simulink model "IEEE39_IBR_FrequencyControl_Primary_2020b"  (R2020b)
settings: Solver=VariableStepAuto  StartTime=0.0  StopTime=30  RelTol=1e-3
InitFcn:
  | IEEE39data_FrencyControl_primary;
undefined symbols (not defined in the file): Fref, IBR_data, line, Sbase, t_start_disturbance, Vbase
libraries: powerlib x203, powerlib_meascontrol x81, powerlib_extras x27, pid_lib x14
(part 2 of 5)

== system IEEE39_IBR_FrequencyControl_Primary_2020b/Subsystem ==
  Mux : Mux  Inputs=10
  Mux2 : Mux  Inputs=10
  Scope2 : Scope
  Scope3 : Scope
  wires:
  [f10] -> Mux/10
  [f1] -> Mux/1
  [f2] -> Mux/2
  [f3] -> Mux/3
  [f4] -> Mux/4
  [f5] -> Mux/5
  [f6] -> Mux/6
  [f7] -> Mux/7
  [f8] -> Mux/8
  [f9] -> Mux/9
  Mux/1 -> Scope2/1
  [P_GFL1] -> Mux2/1
  Mux2/1 -> Scope3/1
  [P_GFL2] -> Mux2/2
  [P_GFL3] -> Mux2/3
  [P_GFL4] -> Mux2/4
  [P_GFL5] -> Mux2/5
  [P_GFL6] -> Mux2/6
  [P_GFM7] -> Mux2/7
  [P_GFM8] -> Mux2/8
  [P_GFM9] -> Mux2/9
  [P_GFM10] -> Mux2/10

== system IEEE39_IBR_FrequencyControl_Primary_2020b/Bus voltages/V_F_measurements30 ==
  abc : Inport
  Display16 : Display
      settings: Format=bank
  PLL (3ph) : powerlib_meascontrol/PLL/PLL (3ph)  Fmin=59.5  Par_Init=[0, 60]  ParK=[180, 3200, 1]  TcD=1e-4  MaxRateChangeFreq=12  FilterCutOffFreq=25  Ts=1e-5  AGC=on
  tag scope: f1=global, f_B30=global
  wires:
  abc/1 -> PLL (3ph)/1
  PLL (3ph)/1 -> [f1], [f_B30], Display16/1

== system IEEE39_IBR_FrequencyControl_Primary_2020b/Bus voltages/V_F_measurements31 ==
  abc : Inport
  PLL (3ph) : powerlib_meascontrol/PLL/PLL (3ph)  Fmin=59.5  Par_Init=[0, 60]  ParK=[180, 3200, 1]  TcD=1e-4  MaxRateChangeFreq=12  FilterCutOffFreq=25  Ts=1e-5  AGC=on
  tag scope: f2=global, f_B31=global
  wires:
  abc/1 -> PLL (3ph)/1
  PLL (3ph)/1 -> [f2], [f_B31]

== system IEEE39_IBR_FrequencyControl_Primary_2020b/Bus voltages/V_F_measurements32 ==
  abc : Inport
  Display16 : Display
      settings: Format=bank
  PLL (3ph) : powerlib_meascontrol/PLL/PLL (3ph)  Fmin=59.5  Par_Init=[0, 60]  ParK=[180, 3200, 1]  TcD=1e-4  MaxRateChangeFreq=12  FilterCutOffFreq=25  Ts=1e-5  AGC=on
  tag scope: f3=global, f_B32=global
  wires:
  abc/1 -> PLL (3ph)/1
  PLL (3ph)/1 -> [f3], [f_B32], Display16/1

== system IEEE39_IBR_FrequencyControl_Primary_2020b/Bus voltages/V_F_measurements33 ==
  abc : Inport
  Display16 : Display
      settings: Format=bank
  PLL (3ph) : powerlib_meascontrol/PLL/PLL (3ph)  Fmin=59.5  Par_Init=[0, 60]  ParK=[180, 3200, 1]  TcD=1e-4  MaxRateChangeFreq=12  FilterCutOffFreq=25  Ts=1e-5  AGC=on
  tag scope: f4=global, f_B33=global
  wires:
  abc/1 -> PLL (3ph)/1
  PLL (3ph)/1 -> [f_B33], Display16/1, [f4]

== system IEEE39_IBR_FrequencyControl_Primary_2020b/Bus voltages/V_F_measurements34 ==
  abc : Inport
  Display16 : Display
      settings: Format=bank
  PLL (3ph) : powerlib_meascontrol/PLL/PLL (3ph)  Fmin=59.5  Par_Init=[0, 60]  ParK=[180, 3200, 1]  TcD=1e-4  MaxRateChangeFreq=12  FilterCutOffFreq=25  Ts=1e-5  AGC=on
  tag scope: f5=global, f_B34=global
  wires:
  abc/1 -> PLL (3ph)/1
  PLL (3ph)/1 -> [f_B34], Display16/1, [f5]

== system IEEE39_IBR_FrequencyControl_Primary_2020b/Bus voltages/V_F_measurements35 ==
  abc : Inport
  Display16 : Display
      settings: Format=bank
  PLL (3ph) : powerlib_meascontrol/PLL/PLL (3ph)  Fmin=59.5  Par_Init=[0, 60]  ParK=[180, 3200, 1]  TcD=1e-4  MaxRateChangeFreq=12  FilterCutOffFreq=25  Ts=1e-5  AGC=on
  tag scope: f6=global, f_B35=global
  wires:
  abc/1 -> PLL (3ph)/1
  PLL (3ph)/1 -> [f6], [f_B35], Display16/1

== system IEEE39_IBR_FrequencyControl_Primary_2020b/Bus voltages/V_F_measurements36 ==
  abc : Inport
  Display16 : Display
      settings: Format=bank
  PLL (3ph) : powerlib_meascontrol/PLL/PLL (3ph)  Fmin=59.5  Par_Init=[0, 60]  ParK=[180, 3200, 1]  TcD=1e-4  MaxRateChangeFreq=12  FilterCutOffFreq=25  Ts=1e-5  AGC=on
  tag scope: f7=global, f_B36=global
  wires:
  abc/1 -> PLL (3ph)/1
  PLL (3ph)/1 -> [f7], [f_B36], Display16/1

== system IEEE39_IBR_FrequencyControl_Primary_2020b/Bus voltages/V_F_measurements37 ==
  abc : Inport
  Display16 : Display
      settings: Format=bank
  PLL (3ph) : powerlib_meascontrol/PLL/PLL (3ph)  Fmin=59.5  Par_Init=[0, 60]  ParK=[180, 3200, 1]  TcD=1e-4  MaxRateChangeFreq=12  FilterCutOffFreq=25  Ts=1e-5  AGC=on
  tag scope: f8=global, f_B37=global
  wires:
  abc/1 -> PLL (3ph)/1
  PLL (3ph)/1 -> [f8], [f_B37], Display16/1

== system IEEE39_IBR_FrequencyControl_Primary_2020b/Bus voltages/V_F_measurements38 ==
  abc : Inport
  Display16 : Display
      settings: Format=bank
  PLL (3ph) : powerlib_meascontrol/PLL/PLL (3ph)  Fmin=59.5  Par_Init=[0, 60]  ParK=[180, 3200, 1]  TcD=1e-4  MaxRateChangeFreq=12  FilterCutOffFreq=25  Ts=1e-5  AGC=on
  tag scope: f9=global, f_B38=global
  wires:
  abc/1 -> PLL (3ph)/1
  PLL (3ph)/1 -> [f9], [f_B38], Display16/1

== system IEEE39_IBR_FrequencyControl_Primary_2020b/Bus voltages/V_F_measurements39 ==
  abc : Inport
  Display16 : Display
      settings: Format=bank
  PLL (3ph) : powerlib_meascontrol/PLL/PLL (3ph)  Fmin=59.5  Par_Init=[0, 60]  ParK=[180, 3200, 1]  TcD=1e-4  MaxRateChangeFreq=12  FilterCutOffFreq=25  Ts=1e-5  AGC=on
  tag scope: f10=global, f_B39=global
  wires:
  abc/1 -> PLL (3ph)/1
  PLL (3ph)/1 -> [f10], [f_B39], Display16/1

== system IEEE39_IBR_FrequencyControl_Primary_2020b/G1_GFL/PV_PQ3 ==
  Pref : Inport
  Qref : Inport  Port=2
  Fref : Inport  Port=3
  D : Inport  Port=4
  3-phase Instantaneous Active & Reactive Power4 : powerlib_extras/Measurements/3-phase  Instantaneous  Active & Reactive Power
  Controlled Voltage Source : powerlib/Electrical Sources/Controlled Voltage Source  Initialize=off  Source_Type=AC  Amplitude=0  Phase=0  Frequency=60  Measurements=None
  Controlled Voltage Source1 : powerlib/Electrical Sources/Controlled Voltage Source  Initialize=off  Source_Type=AC  Amplitude=0  Phase=-120  Frequency=60  Measurements=None
  Controlled Voltage Source3 : powerlib/Electrical Sources/Controlled Voltage Source  Initialize=off  Source_Type=DC  Amplitude=0  Phase=120  Frequency=60  Measurements=None
  Demux : Demux  Outputs=2
  Freq_Droop : Subsystem
  Ground : powerlib/Elements/Ground  LConnTagsString=a
  Ground1 : powerlib/Elements/Ground  LConnTagsString=a
  L : powerlib/Elements/Three-Phase Series RLC Branch  LConnTagsString=A|B|C  RConnTagsString=A|B|C  BranchType=RL  Resistance=0  Inductance=10e-3  Capacitance=1.0  Measurements=None
  L1 : Constant  Value=10e-3
  Mean : powerlib_meascontrol/Measurements/Mean  Freq=60  Vinit=0  Ts=5e-4
  PLL (3ph) : powerlib_meascontrol/PLL/PLL (3ph)  Fmin=59.5  Par_Init=[0, 60]  ParK=[180, 3200, 1]  TcD=1e-4  MaxRateChangeFreq=12  FilterCutOffFreq=25  Ts=1e-5  AGC=on
  Subsystem2 : Subsystem
  Terminator : Terminator
  Terminator1 : Terminator
  Three-Phase Series RLC Branch : powerlib/Elements/Three-Phase Series RLC Branch  LConnTagsString=A|B|C  RConnTagsString=A|B|C  BranchType=RC  Resistance=1000000  Inductance=1e-3  Capacitance=1000e-6  Measurements=None
  Three-Phase V-I Measurement : powerlib/Measurements/Three-Phase V-I Measurement  VoltageMeasurement=phase-to-ground  SetLabelV=off  LabelV=Vabc  Vpu=off  VpuLL=off  CurrentMeasurement=yes  SetLabelI=off  LabelI=Iabc  Ipu=off  Pbase=1e5  Vbase=380  OutputType=Complex  PhasorSimulation=off  PSBequivalent=0
  Three-Phase V-I Measurement4 : powerlib/Measurements/Three-Phase V-I Measurement  VoltageMeasurement=no  SetLabelV=off  LabelV=u  Vpu=off  VpuLL=off  CurrentMeasurement=yes  SetLabelI=off  LabelI=iFabcp3  Ipu=off  Pbase=100e6  Vbase=500e3  OutputType=Complex  PhasorSimulation=off  PSBequivalent=0
  Unit Delay : UnitDelay  SampleTime=-1  HasFrameUpgradeWarning=on
  Unit Delay1 : UnitDelay  SampleTime=-1  HasFrameUpgradeWarning=on
  Unit Delay2 : UnitDelay  SampleTime=-1  HasFrameUpgradeWarning=on
  PV_BatteryA : PMIOPort  Side=Right
  PV_BatteryB : PMIOPort  Port=2  Side=Right
  PV_BatteryC : PMIOPort  Port=3  Side=Right
  tag scope: P_GFL1=global
  wires:
  Three-Phase V-I Measurement/1 -> 3-phase Instantaneous Active & Reactive Power4/1, PLL (3ph)/1, Subsystem2/1(Vabcp)
  Three-Phase V-I Measurement/2 -> Subsystem2/2(Iabcp), 3-phase Instantaneous Active & Reactive Power4/2
  Mean/1 -> Demux/1
  L1/1 -> Subsystem2/6(L1)
  Three-Phase V-I Measurement4/1 -> Subsystem2/3(IFabcp)
  3-phase Instantaneous Active & Reactive Power4/1 -> Mean/1
  Qref/1 -> Subsystem2/5(Q_set)
  PLL (3ph)/2 -> Terminator/1
  PLL (3ph)/1 -> [Freq]
  Pref/1 -> Freq_Droop/1(Pref)
  Fref/1 -> Freq_Droop/2(Fref)
  [Freq] -> Freq_Droop/3(Freq)
  D/1 -> Freq_Droop/4(D)
  Freq_Droop/1(Pset) -> Subsystem2/4(P_set)
  Subsystem2/1(Va) -> Unit Delay/1
  Unit Delay/1 -> Controlled Voltage Source/1
  Subsystem2/2(Vb) -> Unit Delay1/1
  Unit Delay1/1 -> Controlled Voltage Source1/1
  Subsystem2/3(Vc) -> Unit Delay2/1
  Unit Delay2/1 -> Controlled Voltage Source3/1
  Demux/1 -> [P_GFL1]
  Demux/2 -> Terminator1/1
  connections:
  Three-Phase V-I Measurement/LConn1 -- Three-Phase Series RLC Branch/LConn1 -- L/RConn1
  Three-Phase V-I Measurement/RConn2 -- PV_BatteryB/RConn1
  Three-Phase V-I Measurement/LConn2 -- Three-Phase Series RLC Branch/LConn2 -- L/RConn2
  Three-Phase V-I Measurement4/LConn2 -- Controlled Voltage Source1/RConn1
  Controlled Voltage Source/RConn1 -- Three-Phase V-I Measurement4/LConn1
  Three-Phase V-I Measurement4/LConn3 -- Controlled Voltage Source3/RConn1
  Three-Phase V-I Measurement/LConn3 -- Three-Phase Series RLC Branch/LConn3 -- L/RConn3
  Three-Phase V-I Measurement/RConn3 -- PV_BatteryC/RConn1
  Three-Phase V-I Measurement/RConn1 -- PV_BatteryA/RConn1
  Three-Phase V-I Measurement4/RConn1 -- L/LConn1
  Three-Phase V-I Measurement4/RConn2 -- L/LConn2
  Three-Phase V-I Measurement4/RConn3 -- L/LConn3
  Three-Phase Series RLC Branch/RConn1 -- Ground1/LConn1 -- Three-Phase Series RLC Branch/RConn2 -- Three-Phase Series RLC Branch/RConn3
  Controlled Voltage Source/LConn1 -- Controlled Voltage Source3/LConn1 -- Controlled Voltage Source1/LConn1 -- Ground/LConn1

== system IEEE39_IBR_FrequencyControl_Primary_2020b/G2_GFL/PV_PQ3 ==
  Pref : Inport
  Qref : Inport  Port=2
  Fref : Inport  Port=3
  D : Inport  Port=4
  3-phase Instantaneous Active & Reactive Power4 : powerlib_extras/Measurements/3-phase  Instantaneous  Active & Reactive Power
  Controlled Voltage Source : powerlib/Electrical Sources/Controlled Voltage Source  Initialize=on  Source_Type=AC  Amplitude=391.87  Phase=0  Frequency=60  Measurements=None
  Controlled Voltage Source1 : powerlib/Electrical Sources/Controlled Voltage Source  Initialize=on  Source_Type=AC  Amplitude=391.87  Phase=-120  Frequency=60  Measurements=None
  Controlled Voltage Source3 : powerlib/Electrical Sources/Controlled Voltage Source  Initialize=on  Source_Type=AC  Amplitude=391.87  Phase=120  Frequency=60  Measurements=None
  Demux : Demux  Outputs=2
  Freq_Droop : Subsystem
  Ground : powerlib/Elements/Ground  LConnTagsString=a
  Ground1 : powerlib/Elements/Ground  LConnTagsString=a
  L : powerlib/Elements/Three-Phase Series RLC Branch  LConnTagsString=A|B|C  RConnTagsString=A|B|C  BranchType=RL  Resistance=0  Inductance=10e-3  Capacitance=1.0  Measurements=None
  L1 : Constant  Value=10e-3
  Mean : powerlib_meascontrol/Measurements/Mean  Freq=60  Vinit=0  Ts=5e-4
  PLL (3ph) : powerlib_meascontrol/PLL/PLL (3ph)  Fmin=59.5  Par_Init=[0, 60]  ParK=[180, 3200, 1]  TcD=1e-4  MaxRateChangeFreq=12  FilterCutOffFreq=25  Ts=1e-5  AGC=on
  Subsystem2 : Subsystem
  Terminator : Terminator
  Terminator1 : Terminator
  Three-Phase Series RLC Branch : powerlib/Elements/Three-Phase Series RLC Branch  LConnTagsString=A|B|C  RConnTagsString=A|B|C  BranchType=RC  Resistance=1000000  Inductance=1e-3  Capacitance=10000e-6  Measurements=None
  Three-Phase V-I Measurement : powerlib/Measurements/Three-Phase V-I Measurement  VoltageMeasurement=phase-to-ground  SetLabelV=off  LabelV=Vabc  Vpu=off  VpuLL=off  CurrentMeasurement=yes  SetLabelI=off  LabelI=Iabc  Ipu=off  Pbase=1e5  Vbase=380  OutputType=Complex  PhasorSimulation=off  PSBequivalent=0
  Three-Phase V-I Measurement4 : powerlib/Measurements/Three-Phase V-I Measurement  VoltageMeasurement=no  SetLabelV=off  LabelV=u  Vpu=off  VpuLL=off  CurrentMeasurement=yes  SetLabelI=off  LabelI=iFabcp3  Ipu=off  Pbase=100e6  Vbase=500e3  OutputType=Complex  PhasorSimulation=off  PSBequivalent=0
  Unit Delay : UnitDelay  SampleTime=-1  HasFrameUpgradeWarning=on
  Unit Delay1 : UnitDelay  SampleTime=-1  HasFrameUpgradeWarning=on
  Unit Delay2 : UnitDelay  SampleTime=-1  HasFrameUpgradeWarning=on
  PV_BatteryA : PMIOPort  Side=Right
  PV_BatteryB : PMIOPort  Port=2  Side=Right
  PV_BatteryC : PMIOPort  Port=3  Side=Right
  tag scope: P_GFL2=global
  wires:
  Three-Phase V-I Measurement/1 -> 3-phase Instantaneous Active & Reactive Power4/1, PLL (3ph)/1, Subsystem2/1(Vabcp)
  Three-Phase V-I Measurement/2 -> Subsystem2/2(Iabcp), 3-phase Instantaneous Active & Reactive Power4/2
  L1/1 -> Subsystem2/6(L1)
  Three-Phase V-I Measurement4/1 -> Subsystem2/3(IFabcp)
  3-phase Instantaneous Active & Reactive Power4/1 -> Mean/1
  Qref/1 -> Subsystem2/5(Q_set)
  PLL (3ph)/2 -> Terminator/1
  PLL (3ph)/1 -> [Freq]
  Pref/1 -> Freq_Droop/1(Pref)
  Fref/1 -> Freq_Droop/2(Fref)
  [Freq] -> Freq_Droop/3(Freq)
  D/1 -> Freq_Droop/4(D)
  Freq_Droop/1(Pset) -> Subsystem2/4(P_set)
  Subsystem2/1(Va) -> Unit Delay/1
  Unit Delay/1 -> Controlled Voltage Source/1
  Subsystem2/2(Vb) -> Unit Delay1/1
  Unit Delay1/1 -> Controlled Voltage Source1/1
  Subsystem2/3(Vc) -> Unit Delay2/1
  Unit Delay2/1 -> Controlled Voltage Source3/1
  Demux/2 -> Terminator1/1
  Demux/1 -> [P_GFL2]
  Mean/1 -> Demux/1
  connections:
  Three-Phase V-I Measurement/LConn1 -- Three-Phase Series RLC Branch/LConn1 -- L/RConn1
  Three-Phase V-I Measurement/RConn2 -- PV_BatteryB/RConn1
  Three-Phase V-I Measurement/LConn2 -- Three-Phase Series RLC Branch/LConn2 -- L/RConn2
  Three-Phase V-I Measurement4/LConn2 -- Controlled Voltage Source1/RConn1
  Controlled Voltage Source/RConn1 -- Three-Phase V-I Measurement4/LConn1
  Three-Phase V-I Measurement4/LConn3 -- Controlled Voltage Source3/RConn1
  Three-Phase V-I Measurement/LConn3 -- Three-Phase Series RLC Branch/LConn3 -- L/RConn3
  Three-Phase V-I Measurement/RConn3 -- PV_BatteryC/RConn1
  Three-Phase V-I Measurement/RConn1 -- PV_BatteryA/RConn1
  Three-Phase V-I Measurement4/RConn1 -- L/LConn1
  Three-Phase V-I Measurement4/RConn2 -- L/LConn2
  Three-Phase V-I Measurement4/RConn3 -- L/LConn3
  Three-Phase Series RLC Branch/RConn1 -- Ground1/LConn1 -- Three-Phase Series RLC Branch/RConn2 -- Three-Phase Series RLC Branch/RConn3
  Controlled Voltage Source/LConn1 -- Controlled Voltage Source3/LConn1 -- Controlled Voltage Source1/LConn1 -- Ground/LConn1

== system IEEE39_IBR_FrequencyControl_Primary_2020b/G3_GFL/PV_PQ3 ==
  Pref : Inport
  Qref : Inport  Port=2
  Fref : Inport  Port=3
  D : Inport  Port=4
  3-phase Instantaneous Active & Reactive Power4 : powerlib_extras/Measurements/3-phase  Instantaneous  Active & Reactive Power
  Controlled Voltage Source : powerlib/Electrical Sources/Controlled Voltage Source  Initialize=on  Source_Type=AC  Amplitude=391.87  Phase=0  Frequency=60  Measurements=None
  Controlled Voltage Source1 : powerlib/Electrical Sources/Controlled Voltage Source  Initialize=on  Source_Type=AC  Amplitude=391.87  Phase=-120  Frequency=60  Measurements=None
  Controlled Voltage Source3 : powerlib/Electrical Sources/Controlled Voltage Source  Initialize=on  Source_Type=AC  Amplitude=391.87  Phase=120  Frequency=60  Measurements=None
  Demux : Demux  Outputs=2
  Freq_Droop : Subsystem
  Ground : powerlib/Elements/Ground  LConnTagsString=a
  Ground1 : powerlib/Elements/Ground  LConnTagsString=a
  L : powerlib/Elements/Three-Phase Series RLC Branch  LConnTagsString=A|B|C  RConnTagsString=A|B|C  BranchType=RL  Resistance=0  Inductance=100e-3  Capacitance=1.0  Measurements=None
  L1 : Constant  Value=100e-3
  Mean : powerlib_meascontrol/Measurements/Mean  Freq=60  Vinit=0  Ts=5e-4
  PLL (3ph) : powerlib_meascontrol/PLL/PLL (3ph)  Fmin=59.5  Par_Init=[0, 60]  ParK=[180, 3200, 1]  TcD=1e-4  MaxRateChangeFreq=12  FilterCutOffFreq=25  Ts=1e-5  AGC=on
  Subsystem2 : Subsystem
  Terminator : Terminator
  Terminator1 : Terminator
  Three-Phase Series RLC Branch : powerlib/Elements/Three-Phase Series RLC Branch  LConnTagsString=A|B|C  RConnTagsString=A|B|C  BranchType=RC  Resistance=1000000  Inductance=1e-3  Capacitance=10000e-6  Measurements=None
  Three-Phase V-I Measurement : powerlib/Measurements/Three-Phase V-I Measurement  VoltageMeasurement=phase-to-ground  SetLabelV=off  LabelV=Vabc  Vpu=off  VpuLL=off  CurrentMeasurement=yes  SetLabelI=off  LabelI=Iabc  Ipu=off  Pbase=1e5  Vbase=380  OutputType=Complex  PhasorSimulation=off  PSBequivalent=0
  Three-Phase V-I Measurement4 : powerlib/Measurements/Three-Phase V-I Measurement  VoltageMeasurement=no  SetLabelV=off  LabelV=u  Vpu=off  VpuLL=off  CurrentMeasurement=yes  SetLabelI=off  LabelI=iFabcp3  Ipu=off  Pbase=100e6  Vbase=500e3  OutputType=Complex  PhasorSimulation=off  PSBequivalent=0
  Unit Delay : UnitDelay  SampleTime=-1  HasFrameUpgradeWarning=on
  Unit Delay1 : UnitDelay  SampleTime=-1  HasFrameUpgradeWarning=on
  Unit Delay2 : UnitDelay  SampleTime=-1  HasFrameUpgradeWarning=on
  PV_BatteryA : PMIOPort  Side=Right
  PV_BatteryB : PMIOPort  Port=2  Side=Right
  PV_BatteryC : PMIOPort  Port=3  Side=Right
  tag scope: P_GFL3=global
  wires:
  Three-Phase V-I Measurement/2 -> Subsystem2/2(Iabcp), 3-phase Instantaneous Active & Reactive Power4/2
  L1/1 -> Subsystem2/6(L1)
  Three-Phase V-I Measurement4/1 -> Subsystem2/3(IFabcp)
  3-phase Instantaneous Active & Reactive Power4/1 -> Mean/1
  Qref/1 -> Subsystem2/5(Q_set)
  Pref/1 -> Freq_Droop/1(Pref)
  Fref/1 -> Freq_Droop/2(Fref)
  [Freq] -> Freq_Droop/3(Freq)
  D/1 -> Freq_Droop/4(D)
  Freq_Droop/1(Pset) -> Subsystem2/4(P_set)
  Subsystem2/1(Va) -> Unit Delay/1
  Unit Delay/1 -> Controlled Voltage Source/1
  Subsystem2/2(Vb) -> Unit Delay1/1
  Unit Delay1/1 -> Controlled Voltage Source1/1
  Subsystem2/3(Vc) -> Unit Delay2/1
  Unit Delay2/1 -> Controlled Voltage Source3/1
  Demux/2 -> Terminator1/1
  Demux/1 -> [P_GFL3]
  Mean/1 -> Demux/1
  PLL (3ph)/2 -> Terminator/1
  PLL (3ph)/1 -> [Freq]
  Three-Phase V-I Measurement/1 -> PLL (3ph)/1, 3-phase Instantaneous Active & Reactive Power4/1, Subsystem2/1(Vabcp)
  connections:
  Three-Phase V-I Measurement/LConn1 -- Three-Phase Series RLC Branch/LConn1 -- L/RConn1
  Three-Phase V-I Measurement/RConn2 -- PV_BatteryB/RConn1
  Three-Phase V-I Measurement/LConn2 -- Three-Phase Series RLC Branch/LConn2 -- L/RConn2
  Three-Phase V-I Measurement4/LConn2 -- Controlled Voltage Source1/RConn1
  Controlled Voltage Source/RConn1 -- Three-Phase V-I Measurement4/LConn1
  Three-Phase V-I Measurement4/LConn3 -- Controlled Voltage Source3/RConn1
  Three-Phase V-I Measurement/LConn3 -- Three-Phase Series RLC Branch/LConn3 -- L/RConn3
  Three-Phase V-I Measurement/RConn3 -- PV_BatteryC/RConn1
  Three-Phase V-I Measurement/RConn1 -- PV_BatteryA/RConn1
  Three-Phase V-I Measurement4/RConn1 -- L/LConn1
  Three-Phase V-I Measurement4/RConn2 -- L/LConn2
  Three-Phase V-I Measurement4/RConn3 -- L/LConn3
  Three-Phase Series RLC Branch/RConn1 -- Ground1/LConn1 -- Three-Phase Series RLC Branch/RConn2 -- Three-Phase Series RLC Branch/RConn3
  Controlled Voltage Source/LConn1 -- Controlled Voltage Source3/LConn1 -- Controlled Voltage Source1/LConn1 -- Ground/LConn1

== system IEEE39_IBR_FrequencyControl_Primary_2020b/G4_GFL1/PV_PQ3 ==
  Pref : Inport
  Qref : Inport  Port=2
  Fref : Inport  Port=3
  D : Inport  Port=4
  3-phase Instantaneous Active & Reactive Power4 : powerlib_extras/Measurements/3-phase  Instantaneous  Active & Reactive Power
  Controlled Voltage Source : powerlib/Electrical Sources/Controlled Voltage Source  Initialize=on  Source_Type=AC  Amplitude=391.87  Phase=0  Frequency=60  Measurements=None
  Controlled Voltage Source1 : powerlib/Electrical Sources/Controlled Voltage Source  Initialize=on  Source_Type=AC  Amplitude=391.87  Phase=-120  Frequency=60  Measurements=None
  Controlled Voltage Source3 : powerlib/Electrical Sources/Controlled Voltage Source  Initialize=on  Source_Type=AC  Amplitude=391.87  Phase=120  Frequency=60  Measurements=None
  Demux : Demux  Outputs=2
  Freq_Droop : Subsystem
  Ground : powerlib/Elements/Ground  LConnTagsString=a
  Ground1 : powerlib/Elements/Ground  LConnTagsString=a
  L : powerlib/Elements/Three-Phase Series RLC Branch  LConnTagsString=A|B|C  RConnTagsString=A|B|C  BranchType=RL  Resistance=0  Inductance=10e-3  Capacitance=1.0  Measurements=None
  L1 : Constant  Value=10e-3
  Mean : powerlib_meascontrol/Measurements/Mean  Freq=60  Vinit=0  Ts=5e-4
  PLL (3ph) : powerlib_meascontrol/PLL/PLL (3ph)  Fmin=59.5  Par_Init=[0, 60]  ParK=[180, 3200, 1]  TcD=1e-4  MaxRateChangeFreq=12  FilterCutOffFreq=25  Ts=1e-5  AGC=on
  Subsystem2 : Subsystem
  Terminator : Terminator
  Terminator1 : Terminator
  Three-Phase Series RLC Branch : powerlib/Elements/Three-Phase Series RLC Branch  LConnTagsString=A|B|C  RConnTagsString=A|B|C  BranchType=RC  Resistance=1000000  Inductance=1e-3  Capacitance=100e-6  Measurements=None
  Three-Phase V-I Measurement : powerlib/Measurements/Three-Phase V-I Measurement  VoltageMeasurement=phase-to-ground  SetLabelV=off  LabelV=Vabc  Vpu=off  VpuLL=off  CurrentMeasurement=yes  SetLabelI=off  LabelI=Iabc  Ipu=off  Pbase=1e5  Vbase=380  OutputType=Complex  PhasorSimulation=off  PSBequivalent=0
  Three-Phase V-I Measurement4 : powerlib/Measurements/Three-Phase V-I Measurement  VoltageMeasurement=no  SetLabelV=off  LabelV=u  Vpu=off  VpuLL=off  CurrentMeasurement=yes  SetLabelI=off  LabelI=iFabcp3  Ipu=off  Pbase=100e6  Vbase=500e3  OutputType=Complex  PhasorSimulation=off  PSBequivalent=0
  Unit Delay : UnitDelay  SampleTime=-1  HasFrameUpgradeWarning=on
  Unit Delay1 : UnitDelay  SampleTime=-1  HasFrameUpgradeWarning=on
  Unit Delay2 : UnitDelay  SampleTime=-1  HasFrameUpgradeWarning=on
  PV_BatteryA : PMIOPort  Side=Right
  PV_BatteryB : PMIOPort  Port=2  Side=Right
  PV_BatteryC : PMIOPort  Port=3  Side=Right
  tag scope: P_GFL4=global
  wires:
  Three-Phase V-I Measurement/1 -> 3-phase Instantaneous Active & Reactive Power4/1, PLL (3ph)/1, Subsystem2/1(Vabcp)
  Three-Phase V-I Measurement/2 -> Subsystem2/2(Iabcp), 3-phase Instantaneous Active & Reactive Power4/2
  L1/1 -> Subsystem2/6(L1)
  Three-Phase V-I Measurement4/1 -> Subsystem2/3(IFabcp)
  3-phase Instantaneous Active & Reactive Power4/1 -> Mean/1
  Qref/1 -> Subsystem2/5(Q_set)
  PLL (3ph)/2 -> Terminator/1
  PLL (3ph)/1 -> [Freq]
  Pref/1 -> Freq_Droop/1(Pref)
  Fref/1 -> Freq_Droop/2(Fref)
  [Freq] -> Freq_Droop/3(Freq)
  D/1 -> Freq_Droop/4(D)
  Freq_Droop/1(Pset) -> Subsystem2/4(P_set)
  Subsystem2/1(Va) -> Unit Delay/1
  Unit Delay/1 -> Controlled Voltage Source/1
  Subsystem2/2(Vb) -> Unit Delay1/1
  Unit Delay1/1 -> Controlled Voltage Source1/1
  Subsystem2/3(Vc) -> Unit Delay2/1
  Unit Delay2/1 -> Controlled Voltage Source3/1
  Demux/2 -> Terminator1/1
  Demux/1 -> [P_GFL4]
  Mean/1 -> Demux/1
  connections:
  Three-Phase V-I Measurement/LConn1 -- Three-Phase Series RLC Branch/LConn1 -- L/RConn1
  Three-Phase V-I Measurement/RConn2 -- PV_BatteryB/RConn1
  Three-Phase V-I Measurement/LConn2 -- Three-Phase Series RLC Branch/LConn2 -- L/RConn2
  Three-Phase V-I Measurement4/LConn2 -- Controlled Voltage Source1/RConn1
  Controlled Voltage Source/RConn1 -- Three-Phase V-I Measurement4/LConn1
  Three-Phase V-I Measurement4/LConn3 -- Controlled Voltage Source3/RConn1
  Three-Phase V-I Measurement/LConn3 -- Three-Phase Series RLC Branch/LConn3 -- L/RConn3
  Three-Phase V-I Measurement/RConn3 -- PV_BatteryC/RConn1
  Three-Phase V-I Measurement/RConn1 -- PV_BatteryA/RConn1
  Three-Phase V-I Measurement4/RConn1 -- L/LConn1
  Three-Phase V-I Measurement4/RConn2 -- L/LConn2
  Three-Phase V-I Measurement4/RConn3 -- L/LConn3
  Three-Phase Series RLC Branch/RConn1 -- Ground1/LConn1 -- Three-Phase Series RLC Branch/RConn2 -- Three-Phase Series RLC Branch/RConn3
  Controlled Voltage Source/LConn1 -- Controlled Voltage Source3/LConn1 -- Controlled Voltage Source1/LConn1 -- Ground/LConn1

== system IEEE39_IBR_FrequencyControl_Primary_2020b/G5_GFL/PV_PQ3 ==
  Pref : Inport
  Qref : Inport  Port=2
  Fref : Inport  Port=3
  D : Inport  Port=4
  3-phase Instantaneous Active & Reactive Power4 : powerlib_extras/Measurements/3-phase  Instantaneous  Active & Reactive Power
  Controlled Voltage Source : powerlib/Electrical Sources/Controlled Voltage Source  Initialize=on  Source_Type=AC  Amplitude=391.87  Phase=0  Frequency=60  Measurements=None
  Controlled Voltage Source1 : powerlib/Electrical Sources/Controlled Voltage Source  Initialize=on  Source_Type=AC  Amplitude=391.87  Phase=-120  Frequency=60  Measurements=None
  Controlled Voltage Source3 : powerlib/Electrical Sources/Controlled Voltage Source  Initialize=on  Source_Type=AC  Amplitude=391.87  Phase=120  Frequency=60  Measurements=None
  Demux : Demux  Outputs=2
  Freq_Droop : Subsystem
  Ground : powerlib/Elements/Ground  LConnTagsString=a
  Ground1 : powerlib/Elements/Ground  LConnTagsString=a
  L : powerlib/Elements/Three-Phase Series RLC Branch  LConnTagsString=A|B|C  RConnTagsString=A|B|C  BranchType=RL  Resistance=0  Inductance=100e-3  Capacitance=1.0  Measurements=None
  L1 : Constant  Value=100e-3
  Mean : powerlib_meascontrol/Measurements/Mean  Freq=60  Vinit=0  Ts=5e-4
  PLL (3ph) : powerlib_meascontrol/PLL/PLL (3ph)  Fmin=59.5  Par_Init=[0, 60]  ParK=[180, 3200, 1]  TcD=1e-4  MaxRateChangeFreq=12  FilterCutOffFreq=25  Ts=1e-5  AGC=on
  Subsystem2 : Subsystem
  Terminator : Terminator
  Terminator1 : Terminator
  Three-Phase Series RLC Branch : powerlib/Elements/Three-Phase Series RLC Branch  LConnTagsString=A|B|C  RConnTagsString=A|B|C  BranchType=RC  Resistance=1000000  Inductance=1e-3  Capacitance=100e-6  Measurements=None
  Three-Phase V-I Measurement : powerlib/Measurements/Three-Phase V-I Measurement  VoltageMeasurement=phase-to-ground  SetLabelV=off  LabelV=Vabc  Vpu=off  VpuLL=off  CurrentMeasurement=yes  SetLabelI=off  LabelI=Iabc  Ipu=off  Pbase=1e5  Vbase=380  OutputType=Complex  PhasorSimulation=off  PSBequivalent=0
  Three-Phase V-I Measurement4 : powerlib/Measurements/Three-Phase V-I Measurement  VoltageMeasurement=no  SetLabelV=off  LabelV=u  Vpu=off  VpuLL=off  CurrentMeasurement=yes  SetLabelI=off  LabelI=iFabcp3  Ipu=off  Pbase=100e6  Vbase=500e3  OutputType=Complex  PhasorSimulation=off  PSBequivalent=0
  Unit Delay : UnitDelay  SampleTime=-1  HasFrameUpgradeWarning=on
  Unit Delay1 : UnitDelay  SampleTime=-1  HasFrameUpgradeWarning=on
  Unit Delay2 : UnitDelay  SampleTime=-1  HasFrameUpgradeWarning=on
  PV_BatteryA : PMIOPort  Side=Right
  PV_BatteryB : PMIOPort  Port=2  Side=Right
  PV_BatteryC : PMIOPort  Port=3  Side=Right
  tag scope: P_GFL5=global
  wires:
  Three-Phase V-I Measurement/1 -> 3-phase Instantaneous Active & Reactive Power4/1, PLL (3ph)/1, Subsystem2/1(Vabcp)
  Three-Phase V-I Measurement/2 -> Subsystem2/2(Iabcp), 3-phase Instantaneous Active & Reactive Power4/2
  L1/1 -> Subsystem2/6(L1)
  Three-Phase V-I Measurement4/1 -> Subsystem2/3(IFabcp)
  3-phase Instantaneous Active & Reactive Power4/1 -> Mean/1
  Qref/1 -> Subsystem2/5(Q_set)
  PLL (3ph)/2 -> Terminator/1
  PLL (3ph)/1 -> [Freq]
  Pref/1 -> Freq_Droop/1(Pref)
  Fref/1 -> Freq_Droop/2(Fref)
  [Freq] -> Freq_Droop/3(Freq)
  D/1 -> Freq_Droop/4(D)
  Freq_Droop/1(Pset) -> Subsystem2/4(P_set)
  Subsystem2/1(Va) -> Unit Delay/1
  Unit Delay/1 -> Controlled Voltage Source/1
  Subsystem2/2(Vb) -> Unit Delay1/1
  Unit Delay1/1 -> Controlled Voltage Source1/1
  Subsystem2/3(Vc) -> Unit Delay2/1
  Unit Delay2/1 -> Controlled Voltage Source3/1
  Demux/2 -> Terminator1/1
  Demux/1 -> [P_GFL5]
  Mean/1 -> Demux/1
  connections:
  Three-Phase V-I Measurement/LConn1 -- Three-Phase Series RLC Branch/LConn1 -- L/RConn1
  Three-Phase V-I Measurement/RConn2 -- PV_BatteryB/RConn1
  Three-Phase V-I Measurement/LConn2 -- Three-Phase Series RLC Branch/LConn2 -- L/RConn2
  Three-Phase V-I Measurement4/LConn2 -- Controlled Voltage Source1/RConn1
  Controlled Voltage Source/RConn1 -- Three-Phase V-I Measurement4/LConn1
  Three-Phase V-I Measurement4/LConn3 -- Controlled Voltage Source3/RConn1
  Three-Phase V-I Measurement/LConn3 -- Three-Phase Series RLC Branch/LConn3 -- L/RConn3
  Three-Phase V-I Measurement/RConn3 -- PV_BatteryC/RConn1
  Three-Phase V-I Measurement/RConn1 -- PV_BatteryA/RConn1
  Three-Phase V-I Measurement4/RConn1 -- L/LConn1
  Three-Phase V-I Measurement4/RConn2 -- L/LConn2
  Three-Phase V-I Measurement4/RConn3 -- L/LConn3
  Three-Phase Series RLC Branch/RConn1 -- Ground1/LConn1 -- Three-Phase Series RLC Branch/RConn2 -- Three-Phase Series RLC Branch/RConn3
  Controlled Voltage Source/LConn1 -- Controlled Voltage Source3/LConn1 -- Controlled Voltage Source1/LConn1 -- Ground/LConn1

== system IEEE39_IBR_FrequencyControl_Primary_2020b/G6_GFL/PV_PQ3 ==
  Pref : Inport
  Qref : Inport  Port=2
  Fref : Inport  Port=3
  D : Inport  Port=4
  3-phase Instantaneous Active & Reactive Power4 : powerlib_extras/Measurements/3-phase  Instantaneous  Active & Reactive Power
  Controlled Voltage Source : powerlib/Electrical Sources/Controlled Voltage Source  Initialize=on  Source_Type=AC  Amplitude=391.87  Phase=0  Frequency=60  Measurements=None
  Controlled Voltage Source1 : powerlib/Electrical Sources/Controlled Voltage Source  Initialize=on  Source_Type=AC  Amplitude=391.87  Phase=-120  Frequency=60  Measurements=None
  Controlled Voltage Source3 : powerlib/Electrical Sources/Controlled Voltage Source  Initialize=on  Source_Type=AC  Amplitude=391.87  Phase=120  Frequency=60  Measurements=None
  Demux : Demux  Outputs=2
  Freq_Droop : Subsystem
  Ground : powerlib/Elements/Ground  LConnTagsString=a
  Ground1 : powerlib/Elements/Ground  LConnTagsString=a
  L : powerlib/Elements/Three-Phase Series RLC Branch  LConnTagsString=A|B|C  RConnTagsString=A|B|C  BranchType=RL  Resistance=0  Inductance=10e-3  Capacitance=1.0  Measurements=None
  L1 : Constant  Value=10e-3
  Mean : powerlib_meascontrol/Measurements/Mean  Freq=60  Vinit=0  Ts=5e-4
  PLL (3ph) : powerlib_meascontrol/PLL/PLL (3ph)  Fmin=59.5  Par_Init=[0, 60]  ParK=[180, 3200, 1]  TcD=1e-4  MaxRateChangeFreq=12  FilterCutOffFreq=25  Ts=1e-5  AGC=on
  Scope2 : Scope
  Subsystem2 : Subsystem
  Terminator : Terminator
  Terminator1 : Terminator
  Three-Phase Series RLC Branch : powerlib/Elements/Three-Phase Series RLC Branch  LConnTagsString=A|B|C  RConnTagsString=A|B|C  BranchType=RC  Resistance=1000000  Inductance=1e-3  Capacitance=100e-6  Measurements=None
  Three-Phase V-I Measurement : powerlib/Measurements/Three-Phase V-I Measurement  VoltageMeasurement=phase-to-ground  SetLabelV=off  LabelV=Vabc  Vpu=off  VpuLL=off  CurrentMeasurement=yes  SetLabelI=off  LabelI=Iabc  Ipu=off  Pbase=1e5  Vbase=380  OutputType=Complex  PhasorSimulation=off  PSBequivalent=0
  Three-Phase V-I Measurement4 : powerlib/Measurements/Three-Phase V-I Measurement  VoltageMeasurement=phase-to-ground  SetLabelV=off  LabelV=u  Vpu=off  VpuLL=off  CurrentMeasurement=yes  SetLabelI=off  LabelI=iFabcp3  Ipu=off  Pbase=100e6  Vbase=500e3  OutputType=Complex  PhasorSimulation=off  PSBequivalent=0
  Unit Delay : UnitDelay  SampleTime=-1  HasFrameUpgradeWarning=on
  Unit Delay1 : UnitDelay  SampleTime=-1  HasFrameUpgradeWarning=on
  Unit Delay2 : UnitDelay  SampleTime=-1  HasFrameUpgradeWarning=on
  PV_BatteryA : PMIOPort  Side=Right
  PV_BatteryB : PMIOPort  Port=2  Side=Right
  PV_BatteryC : PMIOPort  Port=3  Side=Right
  tag scope: P_GFL6=global
  wires:
  Three-Phase V-I Measurement/1 -> 3-phase Instantaneous Active & Reactive Power4/1, PLL (3ph)/1, Subsystem2/1(Vabcp)
  Three-Phase V-I Measurement/2 -> Subsystem2/2(Iabcp), 3-phase Instantaneous Active & Reactive Power4/2
  L1/1 -> Subsystem2/6(L1)
  Three-Phase V-I Measurement4/2 -> Subsystem2/3(IFabcp)
  3-phase Instantaneous Active & Reactive Power4/1 -> Mean/1
  Three-Phase V-I Measurement4/1 -> Scope2/1
  Qref/1 -> Subsystem2/5(Q_set)
  PLL (3ph)/2 -> Terminator/1
  PLL (3ph)/1 -> [Freq]
  Pref/1 -> Freq_Droop/1(Pref)
  Fref/1 -> Freq_Droop/2(Fref)
  [Freq] -> Freq_Droop/3(Freq)
  D/1 -> Freq_Droop/4(D)
  Freq_Droop/1(Pset) -> Subsystem2/4(P_set)
  Subsystem2/1(Va) -> Unit Delay/1
  Unit Delay/1 -> Controlled Voltage Source/1
  Subsystem2/2(Vb) -> Unit Delay1/1
  Unit Delay1/1 -> Controlled Voltage Source1/1
  Subsystem2/3(Vc) -> Unit Delay2/1
  Unit Delay2/1 -> Controlled Voltage Source3/1
  Demux/2 -> Terminator1/1
  Demux/1 -> [P_GFL6]
  Mean/1 -> Demux/1
  connections:
  Three-Phase V-I Measurement/LConn1 -- Three-Phase Series RLC Branch/LConn1 -- L/RConn1
  Three-Phase V-I Measurement/RConn2 -- PV_BatteryB/RConn1
  Three-Phase V-I Measurement/LConn2 -- Three-Phase Series RLC Branch/LConn2 -- L/RConn2
  Three-Phase V-I Measurement4/LConn2 -- Controlled Voltage Source1/RConn1
  Controlled Voltage Source/RConn1 -- Three-Phase V-I Measurement4/LConn1
  Three-Phase V-I Measurement4/LConn3 -- Controlled Voltage Source3/RConn1
  Three-Phase V-I Measurement/LConn3 -- Three-Phase Series RLC Branch/LConn3 -- L/RConn3
  Three-Phase V-I Measurement/RConn3 -- PV_BatteryC/RConn1
  Three-Phase V-I Measurement/RConn1 -- PV_BatteryA/RConn1
  Three-Phase V-I Measurement4/RConn1 -- L/LConn1
  Three-Phase V-I Measurement4/RConn2 -- L/LConn2
  Three-Phase V-I Measurement4/RConn3 -- L/LConn3
  Three-Phase Series RLC Branch/RConn1 -- Ground1/LConn1 -- Three-Phase Series RLC Branch/RConn2 -- Three-Phase Series RLC Branch/RConn3
  Controlled Voltage Source/LConn1 -- Controlled Voltage Source3/LConn1 -- Controlled Voltage Source1/LConn1 -- Ground/LConn1

== system IEEE39_IBR_FrequencyControl_Primary_2020b/GFM1/PV_PQ3 ==
  Pref : Inport
  Vref_LL : Inport  Port=2
  Fref : Inport  Port=3
  Initial_phase : Inport  Port=4
  3-phase Instantaneous Active & Reactive Power4 : powerlib_extras/Measurements/3-phase  Instantaneous  Active & Reactive Power
  Controlled Voltage Source : powerlib/Electrical Sources/Controlled Voltage Source  Initialize=on  Source_Type=DC  Amplitude=0  Phase=0  Frequency=60  Measurements=None
  Controlled Voltage Source1 : powerlib/Electrical Sources/Controlled Voltage Source  Initialize=on  Source_Type=DC  Amplitude=0  Phase=-120  Frequency=60  Measurements=None
  Controlled Voltage Source3 : powerlib/Electrical Sources/Controlled Voltage Source  Initialize=on  Source_Type=DC  Amplitude=0  Phase=120  Frequency=60  Measurements=None
  Demux : Demux  Outputs=2
  Freq_Droop : Subsystem
  Ground : powerlib/Elements/Ground  LConnTagsString=a
  Ground1 : powerlib/Elements/Ground  LConnTagsString=a
  L : powerlib/Elements/Three-Phase Series RLC Branch  LConnTagsString=A|B|C  RConnTagsString=A|B|C  BranchType=L  Resistance=1  Inductance=0.01  Capacitance=1.0  Measurements=None
  Mean : powerlib_meascontrol/Measurements/Mean  Freq=60  Vinit=0  Ts=5e-4
  PLL (3ph) : powerlib_meascontrol/PLL/PLL (3ph)  Fmin=59.5  Par_Init=[0, 60]  ParK=[180, 3200, 1]  TcD=1e-4  MaxRateChangeFreq=12  FilterCutOffFreq=25  Ts=1e-5  AGC=on
  Three-Phase Series RLC Branch : powerlib/Elements/Three-Phase Series RLC Branch  LConnTagsString=A|B|C  RConnTagsString=A|B|C  BranchType=C  Resistance=0  Inductance=1e-3  Capacitance=1e-6  Measurements=None
  Three-Phase V-I Measurement : powerlib/Measurements/Three-Phase V-I Measurement  VoltageMeasurement=phase-to-ground  SetLabelV=off  LabelV=Vabc  Vpu=off  VpuLL=off  CurrentMeasurement=yes  SetLabelI=off  LabelI=Iabc  Ipu=off  Pbase=1e5  Vbase=380  OutputType=Complex  PhasorSimulation=off  PSBequivalent=0
  Three-Phase V-I Measurement4 : powerlib/Measurements/Three-Phase V-I Measurement  VoltageMeasurement=phase-to-ground  SetLabelV=off  LabelV=u  Vpu=off  VpuLL=off  CurrentMeasurement=yes  SetLabelI=off  LabelI=iFabcp3  Ipu=off  Pbase=100e6  Vbase=500e3  OutputType=Complex  PhasorSimulation=off  PSBequivalent=0
  Unit Delay : UnitDelay  SampleTime=-1  HasFrameUpgradeWarning=on
  Unit Delay1 : UnitDelay  SampleTime=-1  HasFrameUpgradeWarning=on
  Unit Delay2 : UnitDelay  SampleTime=-1  HasFrameUpgradeWarning=on
  V/F : Subsystem
  PV_BatteryA : PMIOPort  Side=Right
  PV_BatteryB : PMIOPort  Port=2  Side=Right
  PV_BatteryC : PMIOPort  Port=3  Side=Right
  tag scope: P_GFM10=global, fre_GFM1_in=global
  wires:
  Three-Phase V-I Measurement/1 -> 3-phase Instantaneous Active & Reactive Power4/1, V/F/1(vabcb)
  Three-Phase V-I Measurement/2 -> V/F/2(iabcb), 3-phase Instantaneous Active & Reactive Power4/2
  Mean/1 -> Demux/1
  Three-Phase V-I Measurement4/2 -> V/F/3(iFabcb)
  3-phase Instantaneous Active & Reactive Power4/1 -> Mean/1
  Three-Phase V-I Measurement4/1 -> PLL (3ph)/1
  Pref/1 -> Freq_Droop/1(Pref)
  Fref/1 -> Freq_Droop/2(Fref)
  [P_meas] -> Freq_Droop/3(Pmeans)
  Freq_Droop/1(fset) -> V/F/5(f)
  Vref_LL/1 -> V/F/4(Vref_LL)
  Initial_phase/1 -> V/F/6(Init_Phase_degree)
  Unit Delay/1 -> Controlled Voltage Source/1
  V/F/1(Va) -> Unit Delay/1
  Unit Delay1/1 -> Controlled Voltage Source1/1
  V/F/2(Vb) -> Unit Delay1/1
  Unit Delay2/1 -> Controlled Voltage Source3/1
  V/F/3(Vc) -> Unit Delay2/1
  Demux/1 -> [P_GFM10], [P_meas]
  PLL (3ph)/1 -> [fre_GFM1_in]
  connections:
  Three-Phase V-I Measurement/LConn1 -- Three-Phase Series RLC Branch/LConn1 -- L/RConn1
  Three-Phase V-I Measurement/RConn2 -- PV_BatteryB/RConn1
  Three-Phase V-I Measurement/LConn2 -- Three-Phase Series RLC Branch/LConn2 -- L/RConn2
  Three-Phase V-I Measurement4/LConn2 -- Controlled Voltage Source1/RConn1
  Controlled Voltage Source/RConn1 -- Three-Phase V-I Measurement4/LConn1
  Three-Phase V-I Measurement4/LConn3 -- Controlled Voltage Source3/RConn1
  Three-Phase V-I Measurement/LConn3 -- Three-Phase Series RLC Branch/LConn3 -- L/RConn3
  Three-Phase V-I Measurement/RConn3 -- PV_BatteryC/RConn1
  Three-Phase V-I Measurement/RConn1 -- PV_BatteryA/RConn1
  Three-Phase V-I Measurement4/RConn1 -- L/LConn1
  Three-Phase V-I Measurement4/RConn2 -- L/LConn2
  Three-Phase V-I Measurement4/RConn3 -- L/LConn3
  Three-Phase Series RLC Branch/RConn1 -- Ground1/LConn1 -- Three-Phase Series RLC Branch/RConn2 -- Three-Phase Series RLC Branch/RConn3
  Controlled Voltage Source/LConn1 -- Controlled Voltage Source3/LConn1 -- Controlled Voltage Source1/LConn1 -- Ground/LConn1

== system IEEE39_IBR_FrequencyControl_Primary_2020b/GFM2/PV_PQ3 ==
  Pref : Inport
  Vref_LL : Inport  Port=2
  Fref : Inport  Port=3
  Initial_phase : Inport  Port=4
  3-phase Instantaneous Active & Reactive Power4 : powerlib_extras/Measurements/3-phase  Instantaneous  Active & Reactive Power
  Controlled Voltage Source : powerlib/Electrical Sources/Controlled Voltage Source  Initialize=on  Source_Type=DC  Amplitude=0  Phase=0  Frequency=60  Measurements=None
  Controlled Voltage Source1 : powerlib/Electrical Sources/Controlled Voltage Source  Initialize=on  Source_Type=DC  Amplitude=0  Phase=-120  Frequency=60  Measurements=None
  Controlled Voltage Source3 : powerlib/Electrical Sources/Controlled Voltage Source  Initialize=on  Source_Type=DC  Amplitude=0  Phase=120  Frequency=60  Measurements=None
  Demux : Demux  Outputs=2
  Freq_Droop : Subsystem
  Ground : powerlib/Elements/Ground  LConnTagsString=a
  Ground1 : powerlib/Elements/Ground  LConnTagsString=a
  L : powerlib/Elements/Three-Phase Series RLC Branch  LConnTagsString=A|B|C  RConnTagsString=A|B|C  BranchType=L  Resistance=1  Inductance=0.01  Capacitance=1.0  Measurements=None
  Mean : powerlib_meascontrol/Measurements/Mean  Freq=60  Vinit=0  Ts=5e-4
  PLL (3ph) : powerlib_meascontrol/PLL/PLL (3ph)  Fmin=59.5  Par_Init=[0, 60]  ParK=[180, 3200, 1]  TcD=1e-4  MaxRateChangeFreq=12  FilterCutOffFreq=25  Ts=1e-5  AGC=on
  Three-Phase Series RLC Branch : powerlib/Elements/Three-Phase Series RLC Branch  LConnTagsString=A|B|C  RConnTagsString=A|B|C  BranchType=C  Resistance=0  Inductance=1e-3  Capacitance=1e-6  Measurements=None
  Three-Phase V-I Measurement : powerlib/Measurements/Three-Phase V-I Measurement  VoltageMeasurement=phase-to-ground  SetLabelV=off  LabelV=Vabc  Vpu=off  VpuLL=off  CurrentMeasurement=yes  SetLabelI=off  LabelI=Iabc  Ipu=off  Pbase=1e5  Vbase=380  OutputType=Complex  PhasorSimulation=off  PSBequivalent=0
  Three-Phase V-I Measurement4 : powerlib/Measurements/Three-Phase V-I Measurement  VoltageMeasurement=phase-to-ground  SetLabelV=off  LabelV=u  Vpu=off  VpuLL=off  CurrentMeasurement=yes  SetLabelI=off  LabelI=iFabcp3  Ipu=off  Pbase=100e6  Vbase=500e3  OutputType=Complex  PhasorSimulation=off  PSBequivalent=0
  Unit Delay : UnitDelay  SampleTime=-1  HasFrameUpgradeWarning=on
  Unit Delay1 : UnitDelay  SampleTime=-1  HasFrameUpgradeWarning=on
  Unit Delay2 : UnitDelay  SampleTime=-1  HasFrameUpgradeWarning=on
  V/F : Subsystem
  PV_BatteryA : PMIOPort  Side=Right
  PV_BatteryB : PMIOPort  Port=2  Side=Right
  PV_BatteryC : PMIOPort  Port=3  Side=Right
  tag scope: P_GFM9=global, fre_GFM_in=global
  wires:
  Three-Phase V-I Measurement/1 -> 3-phase Instantaneous Active & Reactive Power4/1, V/F/1(vabcb)
  Three-Phase V-I Measurement/2 -> V/F/2(iabcb), 3-phase Instantaneous Active & Reactive Power4/2
  Mean/1 -> Demux/1
  Three-Phase V-I Measurement4/2 -> V/F/3(iFabcb)
  3-phase Instantaneous Active & Reactive Power4/1 -> Mean/1
  Three-Phase V-I Measurement4/1 -> PLL (3ph)/1
  Pref/1 -> Freq_Droop/1(Pref)
  Fref/1 -> Freq_Droop/2(Fref)
  [P_meas] -> Freq_Droop/3(Pmeans)
  Freq_Droop/1(fset) -> V/F/5(f)
  Vref_LL/1 -> V/F/4(Vref_LL)
  Initial_phase/1 -> V/F/6(Init_Phase_degree)
  Unit Delay/1 -> Controlled Voltage Source/1
  V/F/1(Va) -> Unit Delay/1
  Unit Delay1/1 -> Controlled Voltage Source1/1
  V/F/2(Vb) -> Unit Delay1/1
  Unit Delay2/1 -> Controlled Voltage Source3/1
  V/F/3(Vc) -> Unit Delay2/1
  Demux/1 -> [P_GFM9], [P_meas]
  PLL (3ph)/1 -> [fre_GFM_in]
  connections:
  Three-Phase V-I Measurement/LConn1 -- Three-Phase Series RLC Branch/LConn1 -- L/RConn1
  Three-Phase V-I Measurement/RConn2 -- PV_BatteryB/RConn1
  Three-Phase V-I Measurement/LConn2 -- Three-Phase Series RLC Branch/LConn2 -- L/RConn2
  Three-Phase V-I Measurement4/LConn2 -- Controlled Voltage Source1/RConn1
  Controlled Voltage Source/RConn1 -- Three-Phase V-I Measurement4/LConn1
  Three-Phase V-I Measurement4/LConn3 -- Controlled Voltage Source3/RConn1
  Three-Phase V-I Measurement/LConn3 -- Three-Phase Series RLC Branch/LConn3 -- L/RConn3
  Three-Phase V-I Measurement/RConn3 -- PV_BatteryC/RConn1
  Three-Phase V-I Measurement/RConn1 -- PV_BatteryA/RConn1
  Three-Phase V-I Measurement4/RConn1 -- L/LConn1
  Three-Phase V-I Measurement4/RConn2 -- L/LConn2
  Three-Phase V-I Measurement4/RConn3 -- L/LConn3
  Three-Phase Series RLC Branch/RConn1 -- Ground1/LConn1 -- Three-Phase Series RLC Branch/RConn2 -- Three-Phase Series RLC Branch/RConn3
  Controlled Voltage Source/LConn1 -- Controlled Voltage Source3/LConn1 -- Controlled Voltage Source1/LConn1 -- Ground/LConn1

== system IEEE39_IBR_FrequencyControl_Primary_2020b/GFM3/PV_PQ3 ==
  Pref : Inport
  Vref_LL : Inport  Port=2
  Fref : Inport  Port=3
  Initial_phase : Inport  Port=4
  3-phase Instantaneous Active & Reactive Power4 : powerlib_extras/Measurements/3-phase  Instantaneous  Active & Reactive Power
  Controlled Voltage Source : powerlib/Electrical Sources/Controlled Voltage Source  Initialize=on  Source_Type=DC  Amplitude=0  Phase=0  Frequency=60  Measurements=None
  Controlled Voltage Source1 : powerlib/Electrical Sources/Controlled Voltage Source  Initialize=on  Source_Type=DC  Amplitude=0  Phase=-120  Frequency=60  Measurements=None
  Controlled Voltage Source3 : powerlib/Electrical Sources/Controlled Voltage Source  Initialize=on  Source_Type=DC  Amplitude=0  Phase=120  Frequency=60  Measurements=None
  Demux : Demux  Outputs=2
  Freq_Droop : Subsystem
  Ground : powerlib/Elements/Ground  LConnTagsString=a
  Ground1 : powerlib/Elements/Ground  LConnTagsString=a
  L : powerlib/Elements/Three-Phase Series RLC Branch  LConnTagsString=A|B|C  RConnTagsString=A|B|C  BranchType=L  Resistance=1  Inductance=0.01  Capacitance=1.0  Measurements=None
  Mean : powerlib_meascontrol/Measurements/Mean  Freq=60  Vinit=0  Ts=5e-4
  Three-Phase Series RLC Branch : powerlib/Elements/Three-Phase Series RLC Branch  LConnTagsString=A|B|C  RConnTagsString=A|B|C  BranchType=C  Resistance=0  Inductance=1e-3  Capacitance=1e-6  Measurements=None
  Three-Phase V-I Measurement : powerlib/Measurements/Three-Phase V-I Measurement  VoltageMeasurement=phase-to-ground  SetLabelV=off  LabelV=Vabc  Vpu=off  VpuLL=off  CurrentMeasurement=yes  SetLabelI=off  LabelI=Iabc  Ipu=off  Pbase=1e5  Vbase=380  OutputType=Complex  PhasorSimulation=off  PSBequivalent=0
  Three-Phase V-I Measurement4 : powerlib/Measurements/Three-Phase V-I Measurement  VoltageMeasurement=no  SetLabelV=off  LabelV=u  Vpu=off  VpuLL=off  CurrentMeasurement=yes  SetLabelI=off  LabelI=iFabcp3  Ipu=off  Pbase=100e6  Vbase=500e3  OutputType=Complex  PhasorSimulation=off  PSBequivalent=0
  Unit Delay : UnitDelay  SampleTime=-1  HasFrameUpgradeWarning=on
  Unit Delay1 : UnitDelay  SampleTime=-1  HasFrameUpgradeWarning=on
  Unit Delay2 : UnitDelay  SampleTime=-1  HasFrameUpgradeWarning=on
  V/F : Subsystem
  PV_BatteryA : PMIOPort  Side=Right
  PV_BatteryB : PMIOPort  Port=2  Side=Right
  PV_BatteryC : PMIOPort  Port=3  Side=Right
  tag scope: P_GFM8=global
  wires:
  Three-Phase V-I Measurement/1 -> 3-phase Instantaneous Active & Reactive Power4/1, V/F/1(vabcb)
  Three-Phase V-I Measurement/2 -> V/F/2(iabcb), 3-phase Instantaneous Active & Reactive Power4/2
  Mean/1 -> Demux/1
  Three-Phase V-I Measurement4/1 -> V/F/3(iFabcb)
  3-phase Instantaneous Active & Reactive Power4/1 -> Mean/1
  Pref/1 -> Freq_Droop/1(Pref)
  Fref/1 -> Freq_Droop/2(Fref)
  [P_meas] -> Freq_Droop/3(Pmeans)
  Freq_Droop/1(fset) -> V/F/5(f)
  Vref_LL/1 -> V/F/4(Vref_LL)
  Initial_phase/1 -> V/F/6(Init_Phase_degree)
  Unit Delay/1 -> Controlled Voltage Source/1
  V/F/1(Va) -> Unit Delay/1
  Unit Delay1/1 -> Controlled Voltage Source1/1
  V/F/2(Vb) -> Unit Delay1/1
  Unit Delay2/1 -> Controlled Voltage Source3/1
  V/F/3(Vc) -> Unit Delay2/1
  Demux/1 -> [P_GFM8], [P_meas]
  connections:
  Three-Phase V-I Measurement/LConn1 -- Three-Phase Series RLC Branch/LConn1 -- L/RConn1
  Three-Phase V-I Measurement/RConn2 -- PV_BatteryB/RConn1
  Three-Phase V-I Measurement/LConn2 -- Three-Phase Series RLC Branch/LConn2 -- L/RConn2
  Three-Phase V-I Measurement4/LConn2 -- Controlled Voltage Source1/RConn1
  Controlled Voltage Source/RConn1 -- Three-Phase V-I Measurement4/LConn1
  Three-Phase V-I Measurement4/LConn3 -- Controlled Voltage Source3/RConn1
  Three-Phase V-I Measurement/LConn3 -- Three-Phase Series RLC Branch/LConn3 -- L/RConn3
  Three-Phase V-I Measurement/RConn3 -- PV_BatteryC/RConn1
  Three-Phase V-I Measurement/RConn1 -- PV_BatteryA/RConn1
  Three-Phase V-I Measurement4/RConn1 -- L/LConn1
  Three-Phase V-I Measurement4/RConn2 -- L/LConn2
  Three-Phase V-I Measurement4/RConn3 -- L/LConn3
  Three-Phase Series RLC Branch/RConn1 -- Ground1/LConn1 -- Three-Phase Series RLC Branch/RConn2 -- Three-Phase Series RLC Branch/RConn3
  Controlled Voltage Source/LConn1 -- Controlled Voltage Source3/LConn1 -- Controlled Voltage Source1/LConn1 -- Ground/LConn1
